simulink model "Control_system_v1"  (R2024b)
settings: Solver=FixedStepDiscrete  StartTime=0.0  StopTime=100  FixedStep=1  RelTol=1e-3
undefined symbols (not defined in the file): A, B, C, D, I_a, K, L, Vk, Wk, x_eq, y_eq
settings Model: Creator=54238  LastModifiedBy=54238

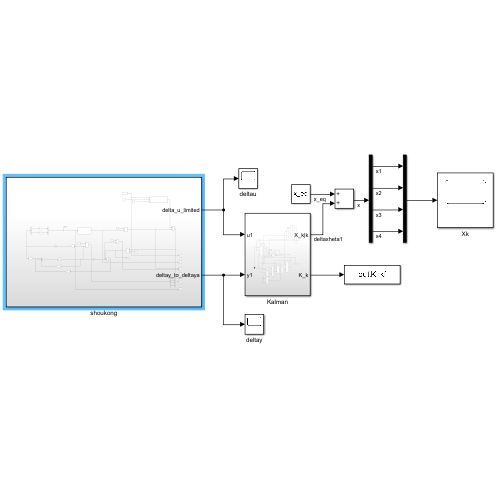
[thumbnail: Simulink's stored preview of the top-level diagram]
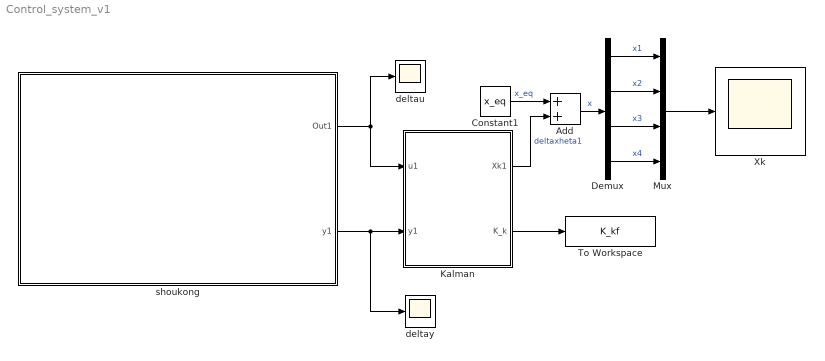
== system Control_system_v1 ==
  Add : Sum
  Constant1 : Constant  Value=x_eq  VectorParams1D=off
  Demux : Demux
  Kalman : Subsystem
  Mux : Mux
  To Workspace : ToWorkspace  VariableName=K_kf  SampleTime=-1
  Xk : Scope
  deltau : Scope
  deltay : Scope
  shoukong : Subsystem
  wires:
  shoukong/2(y1) -> deltay/1, Kalman/2(y1)
  Demux/1 -> Mux/1  "x1"
  Demux/3 -> Mux/3  "x3"
  Demux/2 -> Mux/2  "x2"
  shoukong/1(Out1) -> Kalman/1(u1), deltau/1
  Constant1/1 -> Add/1  "x_eq"
  Kalman/1(Xk1) -> Add/2  "deltaxheta1"
  Add/1 -> Demux/1  "x"
  Demux/4 -> Mux/4  "x4"
  Mux/1 -> Xk/1
  Kalman/2(K_k) -> To Workspace/1

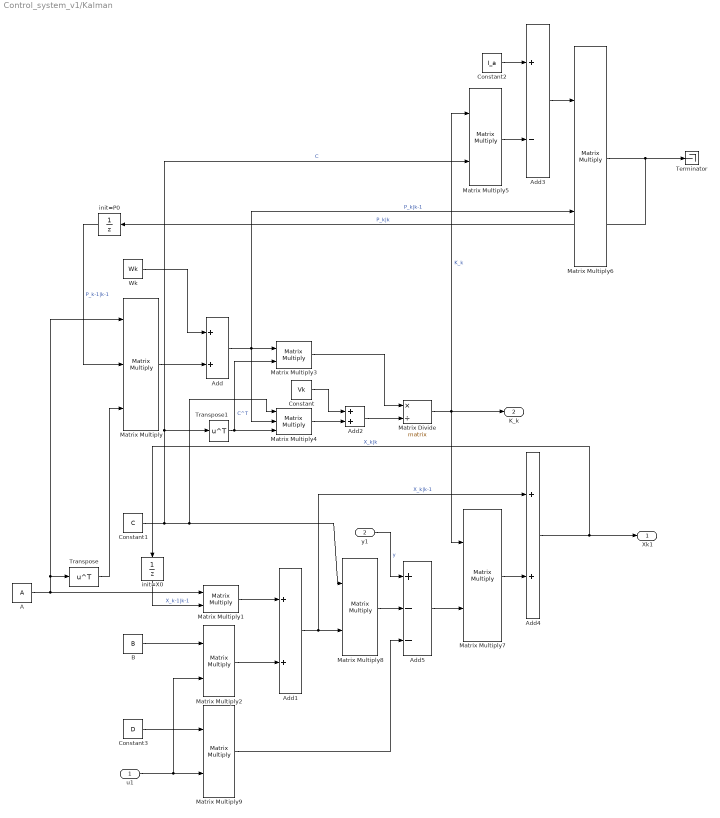
== system Control_system_v1/Kalman ==
  u1 : Inport  PortDimensions=[2,1]
  y1 : Inport  Port=2  PortDimensions=[2,1]
  A : Constant  Value=A
  Add{,1..2,4} (4 alike) : Sum
  Add3 : Sum  Inputs=+-
  Add5 : Sum  Inputs=+--
  B : Constant  Value=B
  Constant : Constant  Value=Vk
  Constant1 : Constant  Value=C
  Constant2 : Constant  Value=I_a
  Constant3 : Constant  Value=D
  Matrix Divide : Product  Inputs=*/  Multiplication=Matrix(*)
  Matrix Multiply : Product  Inputs=3  Multiplication=Matrix(*)
  Matrix Multiply{1..3,5..9} (8 alike) : Product  Multiplication=Matrix(*)
  Matrix Multiply4 : Product  Inputs=3  Multiplication=Matrix(*)
  Terminator : Terminator
  Transpose : Math  Operator=transpose  SignedPower=on  RndMeth=Zero
  Transpose1 : Math  Operator=transpose
  Wk : Constant  Value=Wk
  init=P0 : UnitDelay  SampleTime=-1  StateName=p0  HasFrameUpgradeWarning=on
  init=X0 : UnitDelay  InitialCondition=[5;5;2.044;1.399]  SampleTime=-1  HasFrameUpgradeWarning=on
  Xk1 : Outport  PortDimensions=[4,1]
  K_k : Outport  Port=2
  wires:
  Matrix Multiply2/1 -> Add1/2
  Add5/1 -> Matrix Multiply7/2
  Matrix Multiply6/1 -> Terminator/1, init=P0/1  "P_k|k"
  Constant1/1 -> Matrix Multiply4/1, Matrix Multiply8/1, Matrix Multiply5/2, Transpose1/1  "C"
  Add4/1 -> Xk1/1, init=X0/1  "X_k|k"
  Constant/1 -> Add2/1
  A/1 -> Matrix Multiply/1, Transpose/1, Matrix Multiply1/1
  Add1/1 -> Matrix Multiply8/2, Add4/1  "X_k|k-1"
  Constant2/1 -> Add3/1
  Add/1 -> Matrix Multiply3/1, Matrix Multiply4/2, Matrix Multiply6/2  "P_k|k-1"
  Add3/1 -> Matrix Multiply6/1
  init=X0/1 -> Matrix Multiply1/2  "X_k-1|k-1"
  Transpose/1 -> Matrix Multiply/3
  Matrix Multiply7/1 -> Add4/2
  init=P0/1 -> Matrix Multiply/2  "P_k-1|k-1"
  Matrix Multiply/1 -> Add/2
  Transpose1/1 -> Matrix Multiply4/3, Matrix Multiply3/2  "C^T"
  Wk/1 -> Add/1
  y1/1 -> Add5/1  "y"
  Matrix Multiply5/1 -> Add3/2
  Matrix Divide/1 -> Matrix Multiply5/1, K_k/1, Matrix Multiply7/1  "K_k"
  u1/1 -> Matrix Multiply2/2, Matrix Multiply9/2
  Matrix Multiply1/1 -> Add1/1
  Add2/1 -> Matrix Divide/2
  Matrix Multiply4/1 -> Add2/2
  Constant3/1 -> Matrix Multiply9/1
  Matrix Multiply8/1 -> Add5/2
  B/1 -> Matrix Multiply2/1
  Matrix Multiply9/1 -> Add5/3
  Matrix Multiply3/1 -> Matrix Divide/1

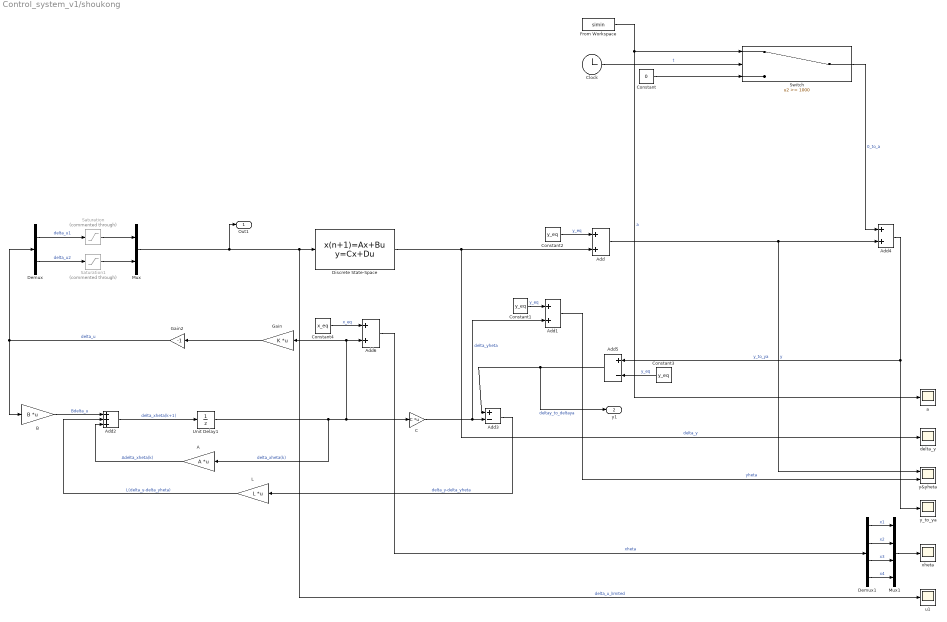
== system Control_system_v1/shoukong ==
  A : Gain  Gain=A  Multiplication=Matrix(K*u)
  Add{,1,4,6} (4 alike) : Sum
  Add2 : Sum  Inputs=+++
  Add3 : Sum  Inputs=+-
  Add5 : Sum  Inputs=+-
  B : Gain  Gain=B  Multiplication=Matrix(K*u)
  C : Gain  Gain=C  Multiplication=Matrix(K*u)
  Clock : Clock
  Constant : Constant  Value=0
  Constant1 : Constant  Value=y_eq  VectorParams1D=off
  Constant2 : Constant  Value=y_eq  VectorParams1D=off
  Constant3 : Constant  Value=y_eq  VectorParams1D=off
  Constant4 : Constant  Value=x_eq  VectorParams1D=off
  Demux : Demux  Outputs=2
  Demux1 : Demux
  Discrete State-Space : DiscreteStateSpace  A=A  B=B  C=C  D=[0 0;0 0]  InitialCondition=[0.5 0.5 0.1 0.1]  SampleTime=-1
  From Workspace : FromWorkspace  VariableName=simin  SampleTime=-1
  Gain : Gain  Gain=K  Multiplication=Matrix(K*u)
  Gain2 : Gain  Gain=-1
  L : Gain  Gain=L  Multiplication=Matrix(K*u)
  Mux : Mux  Inputs=2
  Mux1 : Mux
  Saturation : Saturate  Commented=through  UpperLimit=0.999  LowerLimit=-0.999
  Saturation1 : Saturate  Commented=through  UpperLimit=1.005  LowerLimit=-1.005
  Switch : Switch  Threshold=1000  SaturateOnIntegerOverflow=off  InputSameDT=off
  Unit Delay1 : UnitDelay  SampleTime=-1  HasFrameUpgradeWarning=on
  a : Scope
  delta_y : Scope
  u1 : Scope
  xheta : Scope
  y&yheta : Scope  NumInputPorts=2
  y_to_ya : Scope
  Out1 : Outport  PortDimensions=[2,1]
  y1 : Outport  Port=2  PortDimensions=[2,1]
  wires:
  Add3/1 -> L/1  "delta_y-delta_yheta"
  B/1 -> Add2/1  "Bdelta_u"
  C/1 -> Add1/2, Add3/2  "delta_yheta"
  A/1 -> Add2/3  "Adelta_xheta(k)"
  From Workspace/1 -> Switch/1, a/1  "a"
  Add2/1 -> Unit Delay1/1  "delta_xheta(k+1)"
  Clock/1 -> Switch/2  "t"
  Discrete State-Space/1 -> delta_y/1, Add/2  "delta_y"
  Gain2/1 -> Demux/1, B/1  "delta_u"
  Gain/1 -> Gain2/1
  Unit Delay1/1 -> Add6/2, Gain/1, C/1, A/1  "delta_xheta(k)"
  L/1 -> Add2/2  "L(delta_y-delta_yheta)"
  Constant/1 -> Switch/3
  Switch/1 -> Add4/1  "0_to_a"
  Add4/1 -> Add5/1, y_to_ya/1  "y_to_ya"
  Constant2/1 -> Add/1  "y_eq"
  Add/1 -> y&yheta/1, Add4/2  "y"
  Constant1/1 -> Add1/1  "y_eq"
  Add1/1 -> y&yheta/2  "yheta"
  Constant3/1 -> Add5/2  "y_eq"
  Add5/1 -> y1/1, Add3/1  "deltay_to_deltaya"
  Constant4/1 -> Add6/1  "x_eq"
  Add6/1 -> Demux1/1  "xheta"
  Demux/1 -> Saturation/1  "delta_u1"
  Demux/2 -> Saturation1/1  "delta_u2"
  Saturation1/1 -> Mux/2
  Saturation/1 -> Mux/1
  Mux/1 -> Out1/1, u1/1, Discrete State-Space/1  "delta_u_limited"
  Demux1/1 -> Mux1/1  "x1"
  Demux1/4 -> Mux1/4  "x4"
  Demux1/3 -> Mux1/3  "x3"
  Mux1/1 -> xheta/1
  Demux1/2 -> Mux1/2  "x2"
